simulink model "mVarBus"
settings: Solver=FixedStepDiscrete  StartTime=0.0  StopTime=10.0  RelTol=1e-3
PreLoadFcn:
  | load mvardims_bus3.mat;
CloseFcn:
  | clear a b c d e;
settings Model: ExtModeAutoUpdateStatusClock=off  Creator=djia  LastModifiedBy=hungdang
settings DataIOCC: LimitDataPoints=on  SaveFormat=StructureWithTime  SignalLoggingSaveFormat=ModelDataLogs  SaveTime=off  ReturnWorkspaceOutputs=off
settings OptimizationCC: ExpressionDepthLimit=2147483647  InitFltsAndDblsToZero=on  EfficientMapNaN2IntZero=off  OptimizeModelRefInitCode=on  LifeSpan=1  SimCompilerOptimization=Off
settings DebuggingCC: UnderspecifiedInitializationDetection=Classic  MergeDetectMultiDrivingBlocksExec=none  SignalResolutionControl=TryResolveAllWithWarning  SolverPrmCheckMsg=warning  FcnCallInpInsideContextMsg=UseLocalSettings  FrameProcessingCompatibilityMsg=warning  StateNameClashWarn=warning  SFUnexpectedBacktrackingDiag=warning  SFNoUnconditionalDefaultTransitionDiag=warning
settings HardwareCC: ProdBitPerPointer=32  ProdLargestAtomicFloat=None  ProdIntDivRoundTo=Undefined  ProdEndianess=Unspecified  ProdWordSize=32  ProdHWDeviceType=32-bit Generic
settings ModelReferenceCC: PropagateVarSize=During execution  PropagateSignalLabelsOutOfModel=off
settings SFSimCC: SimUseLocalCustomCode=off
settings RTWCC: SystemTargetFile=ert.tlc  TemplateMakefile=ert_default_tmf  Description=Real-Time Workshop Embedded Coder (no auto configuration)  RetainRTWFile=on  ProcessScript=ert_make_rtw_hook  RTWUseLocalCustomCode=off  RTWCompilerOptimization=Off
settings CodeAppCC: IgnoreCustomStorageClasses=off  MaxIdLength=63  CustomSymbolStrType=$N$R$M
settings ERTTargetCC: CodeReplacementLibrary=ANSI_C  MultiwordLength=2048  GenerateSampleERTMain=on  MatFileLogging=on  InlinedParameterPlacement=NonHierarchical  ERTCustomFileTemplate=example_file_process.tlc  ConvertIfToSwitch=off  SuppressUnreachableDefaultCases=off

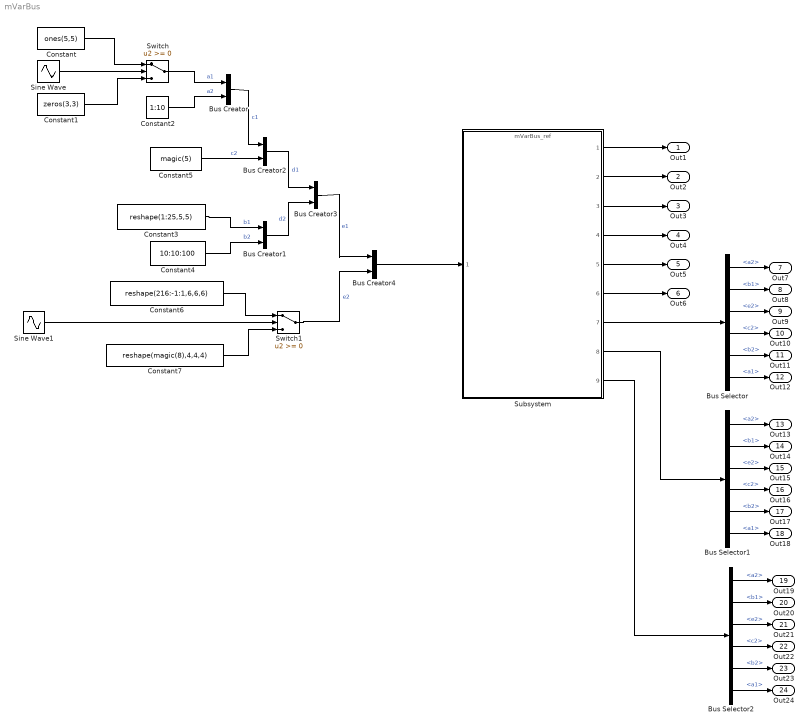
== system mVarBus ==
  Bus Creator : BusCreator  Inputs=2  OutDataTypeStr=Bus: a  NonVirtualBus=on
  Bus Creator1 : BusCreator  Inputs=2  OutDataTypeStr=Bus: b  NonVirtualBus=on
  Bus Creator2 : BusCreator  Inputs=2  OutDataTypeStr=Bus: c  NonVirtualBus=on
  Bus Creator3 : BusCreator  Inputs=2  OutDataTypeStr=Bus: d  NonVirtualBus=on
  Bus Creator4 : BusCreator  Inputs=2  OutDataTypeStr=Bus: e  NonVirtualBus=on
  Bus Selector : BusSelector  OutputSignals=e1.d1.c1.a2,e1.d2.b1,e2,e1.d1.c2,e1.d2.b2,e1.d1.c1.a1
  Bus Selector1 : BusSelector  OutputSignals=e1.d1.c1.a2,e1.d2.b1,e2,e1.d1.c2,e1.d2.b2,e1.d1.c1.a1
  Bus Selector2 : BusSelector  OutputSignals=e1.d1.c1.a2,e1.d2.b1,e2,e1.d1.c2,e1.d2.b2,e1.d1.c1.a1
  Constant : Constant  Value=ones(5,5)
  Constant1 : Constant  Value=zeros(3,3)
  Constant2 : Constant  Value=1:10
  Constant3 : Constant  Value=reshape(1:25,5,5)
  Constant4 : Constant  Value=10:10:100
  Constant5 : Constant  Value=magic(5)
  Constant6 : Constant  Value=reshape(216:-1:1,6,6,6)
  Constant7 : Constant  Value=reshape(magic(8),4,4,4)
  Sine Wave : Sin  SampleTime=.2
  Sine Wave1 : Sin  SampleTime=.2
  Subsystem : ModelReference  ModelNameDialog=mVarBus_ref  ModelReferenceVersion=1.83  CopyOfModelName=mVarBus_ref  DefaultDataLogging=off
  Switch : Switch  AllowDiffInputSizes=on
  Switch1 : Switch  AllowDiffInputSizes=on
  Out1 : Outport
  Out2 : Outport  Port=2
  Out3 : Outport  Port=3
  Out4 : Outport  Port=4
  Out5 : Outport  Port=5
  Out6 : Outport  Port=6
  Out7 : Outport  Port=7
  Out8 : Outport  Port=8
  Out9 : Outport  Port=9
  Out10 : Outport  Port=10
  Out11 : Outport  Port=11
  Out12 : Outport  Port=12
  Out13 : Outport  Port=13
  Out14 : Outport  Port=14
  Out15 : Outport  Port=15
  Out16 : Outport  Port=16
  Out17 : Outport  Port=17
  Out18 : Outport  Port=18
  Out19 : Outport  Port=19
  Out20 : Outport  Port=20
  Out21 : Outport  Port=21
  Out22 : Outport  Port=22
  Out23 : Outport  Port=23
  Out24 : Outport  Port=24
  wires:
  Subsystem/1 -> Out1/1
  Switch/1 -> Bus Creator/1  "a1"
  Constant/1 -> Switch/1
  Constant1/1 -> Switch/3
  Constant2/1 -> Bus Creator/2  "a2"
  Sine Wave/1 -> Switch/2
  Constant4/1 -> Bus Creator1/2  "b2"
  Bus Creator/1 -> Bus Creator2/1  "c1"
  Constant5/1 -> Bus Creator2/2  "c2"
  Bus Creator2/1 -> Bus Creator3/1  "d1"
  Bus Creator1/1 -> Bus Creator3/2  "d2"
  Constant6/1 -> Switch1/1
  Constant7/1 -> Switch1/3
  Sine Wave1/1 -> Switch1/2
  Bus Creator3/1 -> Bus Creator4/1  "e1"
  Switch1/1 -> Bus Creator4/2  "e2"
  Constant3/1 -> Bus Creator1/1  "b1"
  Bus Creator4/1 -> Subsystem/1
  Subsystem/2 -> Out2/1
  Subsystem/3 -> Out3/1
  Subsystem/4 -> Out4/1
  Subsystem/5 -> Out5/1
  Subsystem/6 -> Out6/1
  Bus Selector/1 -> Out7/1  "<a2>"
  Bus Selector/2 -> Out8/1  "<b1>"
  Bus Selector/3 -> Out9/1  "<e2>"
  Bus Selector/4 -> Out10/1  "<c2>"
  Bus Selector/5 -> Out11/1  "<b2>"
  Bus Selector/6 -> Out12/1  "<a1>"
  Subsystem/7 -> Bus Selector/1
  Bus Selector1/1 -> Out13/1  "<a2>"
  Bus Selector1/2 -> Out14/1  "<b1>"
  Bus Selector1/3 -> Out15/1  "<e2>"
  Bus Selector1/4 -> Out16/1  "<c2>"
  Bus Selector1/5 -> Out17/1  "<b2>"
  Bus Selector1/6 -> Out18/1  "<a1>"
  Subsystem/8 -> Bus Selector1/1
  Bus Selector2/1 -> Out19/1  "<a2>"
  Bus Selector2/2 -> Out20/1  "<b1>"
  Bus Selector2/3 -> Out21/1  "<e2>"
  Bus Selector2/4 -> Out22/1  "<c2>"
  Bus Selector2/5 -> Out23/1  "<b2>"
  Bus Selector2/6 -> Out24/1  "<a1>"
  Subsystem/9 -> Bus Selector2/1
